simulink model "ME322_Exercise_2_Prelab_Review_Simulink"  (R2024a)
settings: Solver=VariableStepAuto  StartTime=0.0  StopTime=10.0  RelTol=1e-3
undefined symbols (not defined in the file): b, k, m
settings Model: Creator=clbonney  LastModifiedBy=clbonney

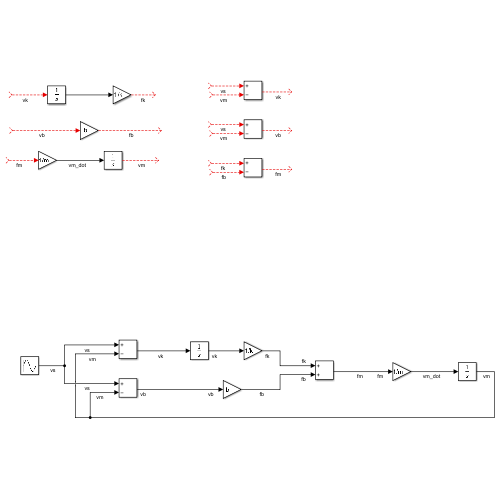
[thumbnail: Simulink's stored preview of the top-level diagram]
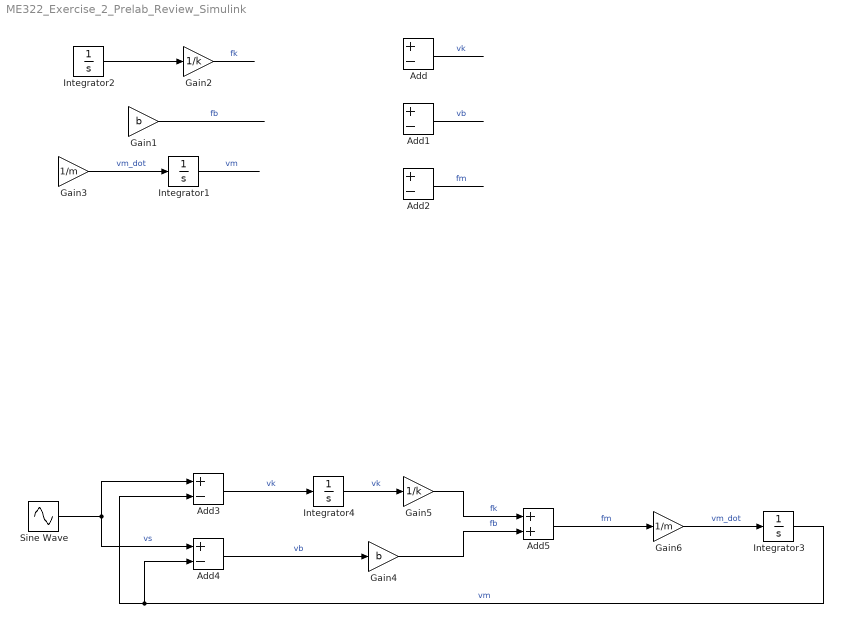
== system ME322_Exercise_2_Prelab_Review_Simulink ==
  Add{,1..4} (5 alike) : Sum  Inputs=+-
  Add5 : Sum
  Gain1 : Gain  Gain=b
  Gain2 : Gain  Gain=1/k
  Gain3 : Gain  Gain=1/m
  Gain4 : Gain  Gain=b
  Gain5 : Gain  Gain=1/k
  Gain6 : Gain  Gain=1/m
  Integrator{1..4} (4 alike) : Integrator
  Sine Wave : Sin  SampleTime=0
  wires:
  Gain1/1 -> ?  "fb"
  ? -> Gain1/1  "vb"
  Gain2/1 -> ?  "fk"
  Integrator2/1 -> Gain2/1
  ? -> Integrator2/1  "vk"
  Gain3/1 -> Integrator1/1  "vm_dot"
  Integrator1/1 -> ?  "vm"
  ? -> Gain3/1  "fm"
  ? -> Add/2  "vm"
  ? -> Add/1  "vs"
  Add/1 -> ?  "vk"
  Add1/1 -> ?  "vb"
  ? -> Add1/1  "vs"
  ? -> Add1/2  "vm"
  ? -> Add2/2  "fb"
  ? -> Add2/1  "fk"
  Add2/1 -> ?  "fm"
  Add3/1 -> Integrator4/1  "vk"
  Add5/1 -> Gain6/1  "fm"
  Integrator3/1 -> Add4/2, Add3/2  "vm"
  Gain6/1 -> Integrator3/1  "vm_dot"
  Integrator4/1 -> Gain5/1  "vk"
  Add4/1 -> Gain4/1  "vb"
  Gain4/1 -> Add5/2  "fb"
  Sine Wave/1 -> Add4/1, Add3/1  "vs"
  Gain5/1 -> Add5/1  "fk"
